simulink model "quadModel"  (R2025b)
settings: Solver=VariableStepAuto  StartTime=0.0  StopTime=10.0  RelTol=1e-3
settings Model: Creator=deepa  LastModifiedBy=deepa

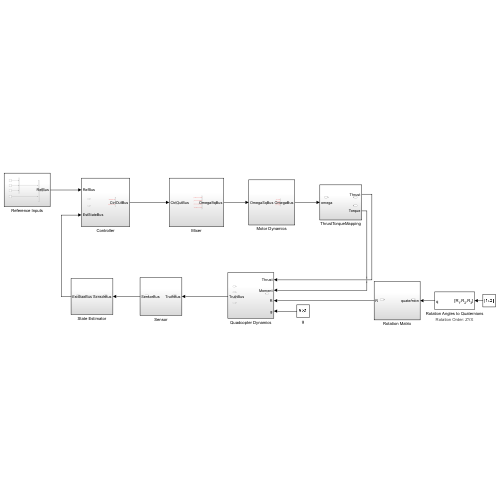
[thumbnail: Simulink's stored preview of the top-level diagram]
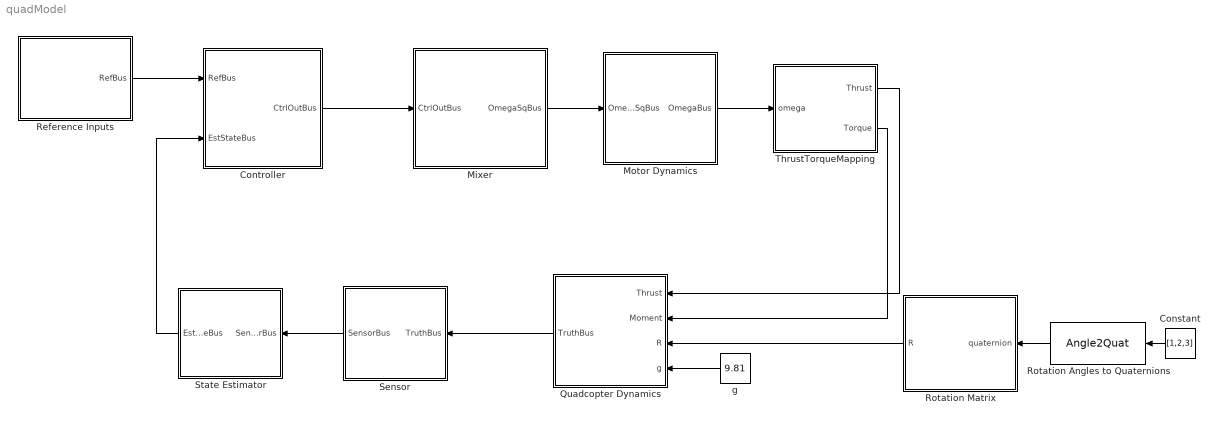
== system quadModel ==
  Constant : Constant  Value=[1,2,3]
  Controller : Subsystem
  Mixer : Subsystem
  Motor Dynamics : Subsystem
  Quadcopter Dynamics : Subsystem
  Reference Inputs : Subsystem
  Rotation Angles to Quaternions : Angle2Quat
      settings: AttributesFormatString=Rotation Order: %<rotationOrder>
  Rotation Matrix : Subsystem
  Sensor : Subsystem
  State Estimator : Subsystem
  ThrustTorqueMapping : Subsystem
  g : Constant  Value=9.81
  wires:
  Mixer/1(OmegaSqBus) -> Motor Dynamics/1(OmegaSqBus)
  Motor Dynamics/1(OmegaBus) -> ThrustTorqueMapping/1(omega)
  Rotation Angles to Quaternions/1 -> Rotation Matrix/1(quaternion)
  Sensor/1(SensorBus) -> State Estimator/1(SensorBus)
  State Estimator/1(EstStaeBus) -> Controller/2(EstStateBus)
  Reference Inputs/1(RefBus) -> Controller/1(RefBus)
  Controller/1(CtrlOutBus) -> Mixer/1(CtrlOutBus)
  Quadcopter Dynamics/1(TruthBus) -> Sensor/1(TruthBus)
  g/1 -> Quadcopter Dynamics/4(g)
  Rotation Matrix/1(R) -> Quadcopter Dynamics/3(R)
  ThrustTorqueMapping/1(Thrust) -> Quadcopter Dynamics/1(Thrust)
  ThrustTorqueMapping/2(Torque) -> Quadcopter Dynamics/2(Moment)
  Constant/1 -> Rotation Angles to Quaternions/1

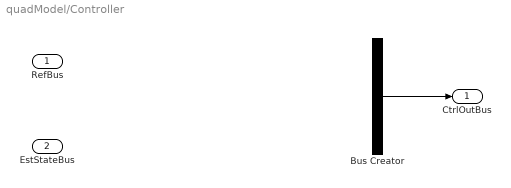
== system quadModel/Controller ==
  RefBus : Inport
  EstStateBus : Inport  Port=2
  Bus Creator : BusCreator  Inputs=2
  CtrlOutBus : Outport
  wires:
  ? -> Bus Creator/1  "F_des(1x1)"
  ? -> Bus Creator/2  "tau_des(3x1)"
  Bus Creator/1 -> CtrlOutBus/1

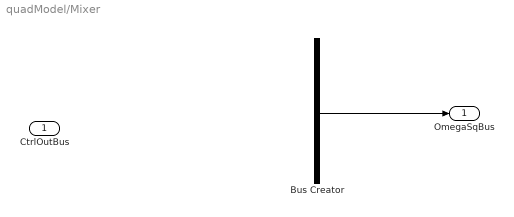
== system quadModel/Mixer ==
  CtrlOutBus : Inport
  Bus Creator : BusCreator  Inputs=4
  OmegaSqBus : Outport
  wires:
  ? -> Bus Creator/1  "w1_sq"
  ? -> Bus Creator/2  "w2_sq"
  ? -> Bus Creator/3  "w3_sq"
  ? -> Bus Creator/4  "w4_sq"
  Bus Creator/1 -> OmegaSqBus/1

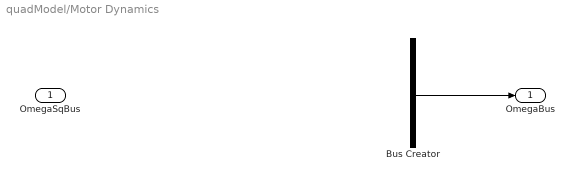
== system quadModel/Motor Dynamics ==
  OmegaSqBus : Inport
  Bus Creator : BusCreator  Inputs=4
  OmegaBus : Outport
  wires:
  ? -> Bus Creator/1  "w1"
  ? -> Bus Creator/2  "w2"
  ? -> Bus Creator/3  "w3"
  ? -> Bus Creator/4  "w4"
  Bus Creator/1 -> OmegaBus/1

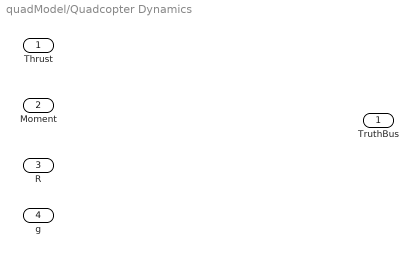
== system quadModel/Quadcopter Dynamics ==
  Thrust : Inport
  Moment : Inport  Port=2
  R : Inport  Port=3
  g : Inport  Port=4
  TruthBus : Outport

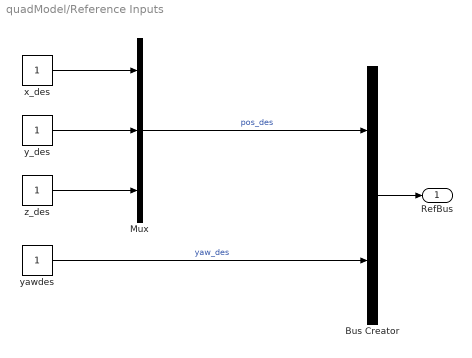
== system quadModel/Reference Inputs ==
  Bus Creator : BusCreator  Inputs=2
  Mux : Mux  Inputs=3
  x_des : Constant
  y_des : Constant
  yawdes : Constant
  z_des : Constant
  RefBus : Outport
  wires:
  x_des/1 -> Mux/1
  y_des/1 -> Mux/2
  z_des/1 -> Mux/3
  Mux/1 -> Bus Creator/1  "pos_des"
  yawdes/1 -> Bus Creator/2  "yaw_des"
  Bus Creator/1 -> RefBus/1

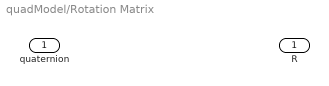
== system quadModel/Rotation Matrix ==
  quaternion : Inport
  R : Outport

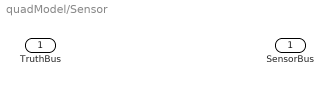
== system quadModel/Sensor ==
  TruthBus : Inport
  SensorBus : Outport

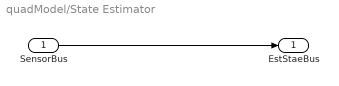
== system quadModel/State Estimator ==
  SensorBus : Inport
  EstStaeBus : Outport
  wires:
  SensorBus/1 -> EstStaeBus/1

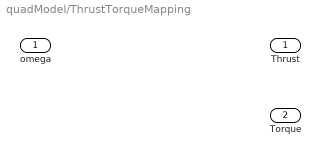
== system quadModel/ThrustTorqueMapping ==
  omega : Inport
  Thrust : Outport
  Torque : Outport  Port=2
